simulink model "uz_inverter_status"  (R2024a)
settings: Solver=FixedStepDiscrete  StartTime=0.0  StopTime=100e-6  RelTol=1e-3  EnableMultiTasking=on
libraries: hdlsllib x14
settings Model: Creator=Geiger  LastModifiedBy=Geiger
settings SolverCC: PositivePriorityOrder=on
settings OptimizationCC: BlockReduction=off  ConditionallyExecuteInputs=off  DefaultParameterBehavior=Inlined  EnhancedBackFolding=on  PassReuseOutputArgsAs=Individual arguments  ZeroExternalMemoryAtStartup=off  ZeroInternalMemoryAtStartup=off  MaxStackSize=64  OptimizeBlockOrder=speed  DifferentSizesBufferReuse=on  OptimizationCustomize=off  EfficientTunableParamExpr=on
settings DebuggingCC: AlgebraicLoopMsg=error  ParameterTunabilityLossMsg=error
settings HardwareCC: ProdBitPerPointer=32  ProdBitPerSizeT=32  ProdBitPerPtrDiffT=32  ProdLargestAtomicFloat=None  ProdIntDivRoundTo=Undefined  ProdEndianess=Unspecified  ProdWordSize=32  ProdHWDeviceType=ASIC/FPGA->ASIC/FPGA  TargetBitPerPointer=64  TargetBitPerSizeT=64  TargetBitPerPtrDiffT=64  TargetLongLongMode=on  TargetIntDivRoundTo=Zero  TargetEndianess=LittleEndian  TargetWordSize=64  TargetHWDeviceType=Custom Processor->MATLAB Host Computer  ProdEqTarget=off
settings ModelReferenceCC: EnableRefExpFcnMdlSchedulingChecks=on
settings SFSimCC: MATLABDynamicMemAlloc=off
settings RTWCC: Description=Embedded Coder  SystemTargetFile=ert.tlc  TemplateMakefile=ert_default_tmf  Toolchain=Linaro AArch64 Linux v6.3.1
settings CodeAppCC: ForceParamTrailComments=on  IgnoreCustomStorageClasses=off  OperatorAnnotations=on  SimulinkDataObjDesc=on  SFDataObjDesc=on  InsertBlockDesc=on
settings ERTTargetCC: InlinedParameterPlacement=NonHierarchical  ERTCustomFileTemplate=example_file_process.tlc

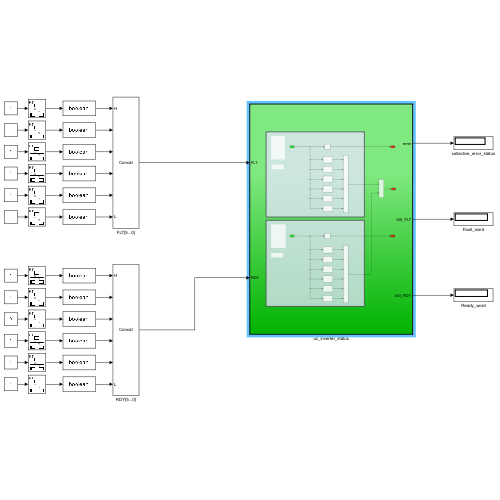
[thumbnail: Simulink's stored preview of the top-level diagram]
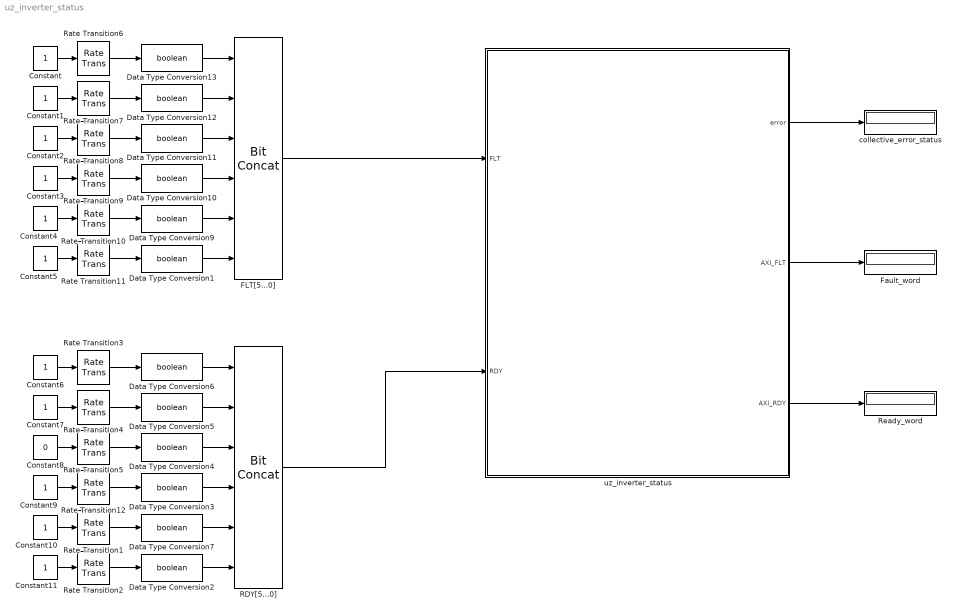
== system uz_inverter_status ==
  Constant{,1..7,9..11} (11 alike) : Constant
  Constant8 : Constant  Value=0
  Data Type Conversion{1..7,9..13} (12 alike) : DataTypeConversion  OutDataTypeStr=boolean  SaturateOnIntegerOverflow=off  RndMeth=Floor
  FLT[5...0] : hdlsllib/Logic and Bit Operations/Bit Concat  numInputs=6
  Fault_word : Display
      settings: Format=binary (Stored Integer)
  RDY[5...0] : hdlsllib/Logic and Bit Operations/Bit Concat  numInputs=6
  Rate Transition{1..12} (12 alike) : RateTransition  OutPortSampleTime=t_clk
  Ready_word : Display
      settings: Format=binary (Stored Integer)
  collective_error_status : Display
  uz_inverter_status : Subsystem  TreatAsAtomicUnit=on
  wires:
  Rate Transition11/1 -> Data Type Conversion1/1
  FLT[5...0]/1 -> uz_inverter_status/1(FLT)
  Rate Transition10/1 -> Data Type Conversion9/1
  Rate Transition6/1 -> Data Type Conversion13/1
  Rate Transition7/1 -> Data Type Conversion12/1
  Data Type Conversion1/1 -> FLT[5...0]/6
  Data Type Conversion12/1 -> FLT[5...0]/2
  Data Type Conversion10/1 -> FLT[5...0]/4
  Rate Transition9/1 -> Data Type Conversion10/1
  Data Type Conversion9/1 -> FLT[5...0]/5
  Data Type Conversion13/1 -> FLT[5...0]/1
  Constant1/1 -> Rate Transition7/1
  Constant4/1 -> Rate Transition10/1
  Constant2/1 -> Rate Transition8/1
  Rate Transition8/1 -> Data Type Conversion11/1
  Constant5/1 -> Rate Transition11/1
  Constant3/1 -> Rate Transition9/1
  Constant/1 -> Rate Transition6/1
  Data Type Conversion11/1 -> FLT[5...0]/3
  Data Type Conversion7/1 -> RDY[5...0]/5
  Constant6/1 -> Rate Transition3/1
  Constant9/1 -> Rate Transition12/1
  Constant11/1 -> Rate Transition2/1
  Data Type Conversion4/1 -> RDY[5...0]/3
  Constant10/1 -> Rate Transition1/1
  Rate Transition5/1 -> Data Type Conversion4/1
  Data Type Conversion6/1 -> RDY[5...0]/1
  Data Type Conversion3/1 -> RDY[5...0]/4
  Data Type Conversion5/1 -> RDY[5...0]/2
  Rate Transition12/1 -> Data Type Conversion3/1
  Rate Transition3/1 -> Data Type Conversion6/1
  Rate Transition1/1 -> Data Type Conversion7/1
  Rate Transition4/1 -> Data Type Conversion5/1
  Data Type Conversion2/1 -> RDY[5...0]/6
  Constant7/1 -> Rate Transition4/1
  Constant8/1 -> Rate Transition5/1
  RDY[5...0]/1 -> uz_inverter_status/2(RDY)
  Rate Transition2/1 -> Data Type Conversion2/1
  uz_inverter_status/2(AXI_FLT) -> Fault_word/1
  uz_inverter_status/3(AXI_RDY) -> Ready_word/1
  uz_inverter_status/1(error) -> collective_error_status/1

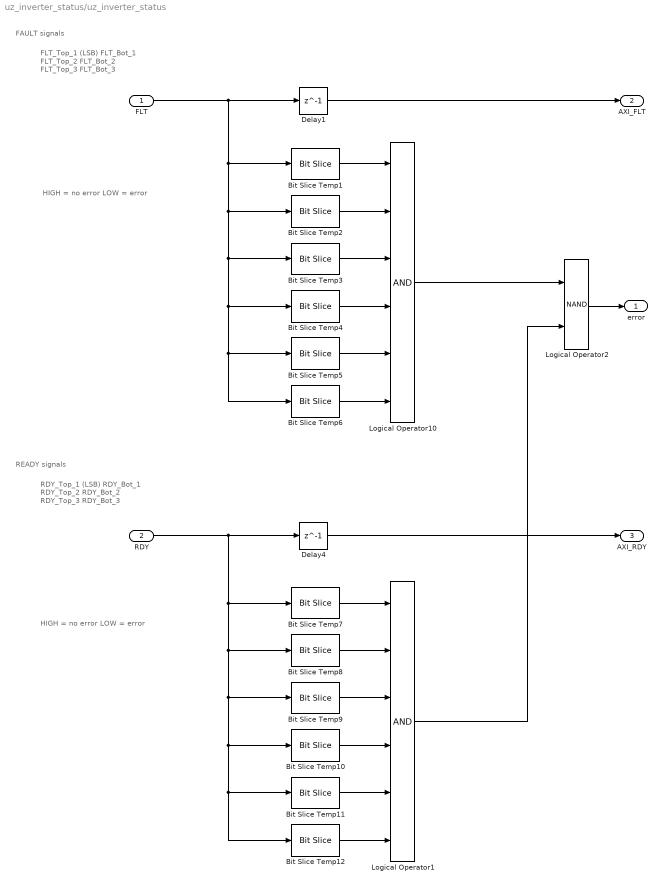
== system uz_inverter_status/uz_inverter_status ==
  note: FLT_Top_1   (LSB)
      |
      | FLT_Bot_1
      |
      | FLT_Top_2
      |
      | FLT_Bot_2
      |
      | FLT_Top_3
      |
      | FLT_Bot_3
  note: FAULT signals
  note: RDY_Top_1   (LSB)
      |
      | RDY_Bot_1
      |
      | RDY_Top_2
      |
      | RDY_Bot_2
      |
      | RDY_Top_3
      |
      | RDY_Bot_3
  note: READY signals
  note: HIGH = no error
      | LOW = error
  note: HIGH = no error
      | LOW = error
  FLT : Inport
  RDY : Inport  Port=2
  Bit Slice Temp1 : hdlsllib/Logic and Bit Operations/Bit Slice  lidx=0  ridx=0
  Bit Slice Temp10 : hdlsllib/Logic and Bit Operations/Bit Slice  lidx=3  ridx=3
  Bit Slice Temp11 : hdlsllib/Logic and Bit Operations/Bit Slice  lidx=4  ridx=4
  Bit Slice Temp12 : hdlsllib/Logic and Bit Operations/Bit Slice  lidx=5  ridx=5
  Bit Slice Temp2 : hdlsllib/Logic and Bit Operations/Bit Slice  lidx=1  ridx=1
  Bit Slice Temp3 : hdlsllib/Logic and Bit Operations/Bit Slice  lidx=2  ridx=2
  Bit Slice Temp4 : hdlsllib/Logic and Bit Operations/Bit Slice  lidx=3  ridx=3
  Bit Slice Temp5 : hdlsllib/Logic and Bit Operations/Bit Slice  lidx=4  ridx=4
  Bit Slice Temp6 : hdlsllib/Logic and Bit Operations/Bit Slice  lidx=5  ridx=5
  Bit Slice Temp7 : hdlsllib/Logic and Bit Operations/Bit Slice  lidx=0  ridx=0
  Bit Slice Temp8 : hdlsllib/Logic and Bit Operations/Bit Slice  lidx=1  ridx=1
  Bit Slice Temp9 : hdlsllib/Logic and Bit Operations/Bit Slice  lidx=2  ridx=2
  Delay1 : Delay  DelayLength=1
  Delay4 : Delay  DelayLength=1
  Logical Operator1 : Logic  Inputs=6  AllPortsSameDT=off  OutDataTypeStr=boolean
  Logical Operator10 : Logic  Inputs=6  AllPortsSameDT=off  OutDataTypeStr=boolean
  Logical Operator2 : Logic  Operator=NAND  AllPortsSameDT=off  OutDataTypeStr=boolean
  error : Outport  VectorParamsAs1DForOutWhenUnconnected=off
  AXI_FLT : Outport  Port=2  PortDimensions=1  VectorParamsAs1DForOutWhenUnconnected=off
  AXI_RDY : Outport  Port=3  PortDimensions=1  VectorParamsAs1DForOutWhenUnconnected=off
  wires:
  Delay1/1 -> AXI_FLT/1
  Delay4/1 -> AXI_RDY/1
  FLT/1 -> Bit Slice Temp6/1, Bit Slice Temp5/1, Bit Slice Temp4/1, Bit Slice Temp3/1, Bit Slice Temp2/1, Bit Slice Temp1/1, Delay1/1
  Bit Slice Temp6/1 -> Logical Operator10/6
  Bit Slice Temp5/1 -> Logical Operator10/5
  Bit Slice Temp4/1 -> Logical Operator10/4
  Bit Slice Temp3/1 -> Logical Operator10/3
  Bit Slice Temp2/1 -> Logical Operator10/2
  Bit Slice Temp1/1 -> Logical Operator10/1
  Bit Slice Temp11/1 -> Logical Operator1/5
  RDY/1 -> Bit Slice Temp12/1, Bit Slice Temp11/1, Bit Slice Temp10/1, Bit Slice Temp9/1, Bit Slice Temp8/1, Bit Slice Temp7/1, Delay4/1
  Bit Slice Temp12/1 -> Logical Operator1/6
  Bit Slice Temp8/1 -> Logical Operator1/2
  Bit Slice Temp9/1 -> Logical Operator1/3
  Bit Slice Temp7/1 -> Logical Operator1/1
  Bit Slice Temp10/1 -> Logical Operator1/4
  Logical Operator10/1 -> Logical Operator2/1
  Logical Operator1/1 -> Logical Operator2/2
  Logical Operator2/1 -> error/1
